simulink model "ofdm_agc_mimo"  (Simulink 7.7)
settings: Solver=VariableStepDiscrete  SolverMode=SingleTasking  StartTime=0.0  StopTime=400  RelTol=1e-3
InitFcn:
  | ofdm_agc_init
StartFcn:
  | ofdm_agc_init
values from neighbouring files (symbols this model uses):
  ltbl = ltbl(2:2049)    [ofdm_agc_init.m]
undefined symbols (not defined in the file or in its folder): gcbh, xlBlockLoadCallback, xlGetNormalizedPeriod
libraries: xbsIndex_r4 x570
(part 1 of 6)
settings Model: Creator=murphpo  LastModifiedBy=murphpo
settings OptimizationCC: InlineParams=on  InitFltsAndDblsToZero=on
settings DebuggingCC: SaveWithParameterizedLinksMsg=none  SignalResolutionControl=TryResolveAllWithWarning  MultiTaskDSMMsg=warning  MultiTaskCondExecSysMsg=none
settings RTWCC: IncludeERTFirstTime=on
settings GRTTargetCC: TargetFcnLib=ansi_tfl_tmw.mat

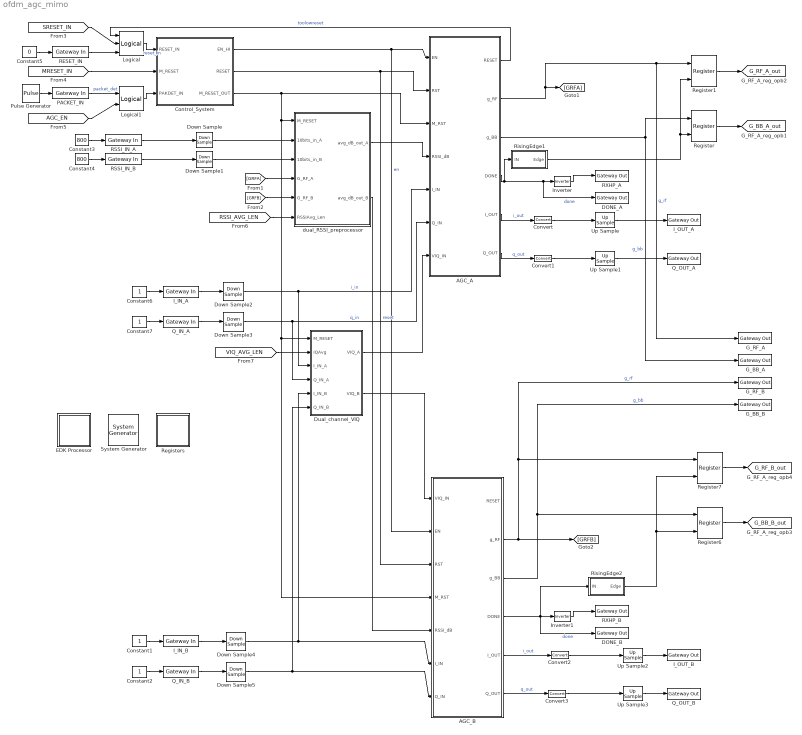
== system ofdm_agc_mimo ==
  " System Generator" : xbsIndex_r4/ System Generator  Tag=genX  SystemSampleTime=-1  xilinxfamily=virtex6  part=xc6vlx130t  speed=-1  package=ff1156  synthesis_tool=XST  clock_wrapper=Clock Enables  directory=./plb46_V6_v0  proj_type=Project Navigator  Synth_file=XST Defaults  Impl_file=ISE Defaults  testbench=off  simulink_period=1  sysclk_period=10  dcm_input_clock_period=100  incr_netlist=off  trim_vbits=Everywhere in SubSystem  dbl_ovrd=According to Block Masks  core_generation=According to Block Masks  run_coregen=off  deprecated_control=off  eval_field=0  block_type=sysgen
      settings: block_version=8.2
  AGC_A : Subsystem
  AGC_B : Subsystem
  Constant{1..2,6..7} (4 alike) : Constant
  Constant3 : Constant  Value=800
  Constant4 : Constant  Value=800
  Constant5 : Constant  Value=0
  Control_System : Subsystem
  Convert{,1..3} (4 alike) : xbsIndex_r4/Convert  gui_display_data_type=Fixed-point  arith_type="Signed  (2's comp)"  n_bits=14  bin_pt=13  float_type=Single  exp_bits=8  fraction_bits=24  quantization=Truncate  overflow=Saturate  en=off  latency=0  dbl_ovrd=off  pipeline=off  block_type=convert
      settings: xl_area=[8 0 0 15 0 0 0]  block_version=VER_STRING_GOES_HERE
  DONE_A : xbsIndex_r4/Gateway Out  inherit_from_input=off  hdl_port=on  timing_constraint=None  locs_specified=off  LOCs={}  UseAsDAC=off  DACChannel='1'  block_type=gatewayout
      settings: infoedit="Gateway out block.  Converts Xilinx fixed point inputs into ouputs of type Simulink integer, double, or fixed point.<P><P>Hardware notes:  In hardware these blocks become top level output ports or are discarded, depending on how they are configured."  xl_area=[0 0 0 0 1 0 0]  block_version=VER_STRING_GOES_HERE
  DONE_B : xbsIndex_r4/Gateway Out  inherit_from_input=off  hdl_port=on  timing_constraint=None  locs_specified=off  LOCs={}  UseAsDAC=off  DACChannel='1'  block_type=gatewayout
      settings: infoedit="Gateway out block.  Converts Xilinx fixed point inputs into ouputs of type Simulink integer, double, or fixed point.<P><P>Hardware notes:  In hardware these blocks become top level output ports or are discarded, depending on how they are configured."  xl_area=[0 0 0 0 1 0 0]  block_version=VER_STRING_GOES_HERE
  Down Sample{,1..5} (6 alike) : xbsIndex_r4/Down Sample  sample_ratio=4  sample_phase="Last Value of Frame  (most efficient)"  en=off  latency=1  dbl_ovrd=off  block_type=dsamp
      Down Sample settings: block_version=8.2.02
      Down Sample1 settings: block_version=8.2.02
      Down Sample2 settings: xl_area=[7 14 0 0 0 0 0]  block_version=VER_STRING_GOES_HERE
      Down Sample3 settings: xl_area=[7 14 0 0 0 0 0]  block_version=VER_STRING_GOES_HERE
      Down Sample4 settings: xl_area=[7 14 0 0 0 0 0]  block_version=VER_STRING_GOES_HERE
      Down Sample5 settings: xl_area=[7 14 0 0 0 0 0]  block_version=VER_STRING_GOES_HERE
  Dual_channel_VIQ : Subsystem
  EDK Processor : Subsystem  LoadFcn=xlBlockLoadCallback(gcbh);  mask(Xilinx EDK Processor Block){mode=EDK pcore generation, xmp=, MemVisToProc=<qt bgcolor="#FFFFFF"><div><img src="C:/Xilinx/13.4/ISE_DS/ISE/sysgen/data/images/registerplus.gif"> &lt;&lt;Bits_w&gt;&gt;<br></div><div><img src="C:/Xilinx/13.4/ISE_DS/ISE/sysgen/data/images/registerplus.gif"> &lt;&lt;GBB_init&gt;&gt;<br></div><div><img src="C:/Xilinx/13.4/ISE_DS/ISE/sysgen/data/images/registerplus.gif"> &lt;&lt;ADJ&gt;&gt;<br></div><div><img src="C:/Xilinx/13.4/ISE_DS/ISE/sysgen/data/images/registerplus.gif"> &lt;&lt;DCO_IIR_Coef_FB&gt;&gt;<br></div><div><img src="C:/Xilinx/13.4/ISE_DS/ISE/sysgen/data/images/registerplus.gif"> &lt;&lt;Thresholds&gt;&gt;<br></div><div><img src="C:/Xilinx/13.4/ISE_DS/ISE/sysgen/data/images/registerplus.gif"> &lt;&lt;Timing&gt;&gt;<br></div><div><img src="C:/Xilinx/13.4/ISE_DS/ISE/sysgen/data/images/registerplus.gif"> &lt;&lt;DCO_IIR_Coef_Gain&gt;&gt;<br></div><div><img src="C:/Xilinx/13.4/ISE_DS/ISE/sysgen/data/images/registerplus.gif"> &lt;&lt;AVG_LEN&gt;&gt;<br></div><div><img src="C:/Xilinx/13.4/ISE_DS/ISE/sysgen/data/images/registerplus.gif"> &lt;&lt;AGC_EN&gt;&gt;<br></div><div><img src="C:/Xilinx/13.4/ISE_DS/ISE/sysgen/data/images/registerplus.gif"> &lt;&lt;DCO_Timing&gt;&gt;<br></div><div><img src="C:/Xilinx/13.4/ISE_DS/ISE/sysgen/data/images/registerplus.gif"> &lt;&lt;T_dB&gt;&gt;<br></div><div><img src="C:/Xilinx/13.4/ISE_DS/ISE/sysgen/data/images/registerplus.gif"> &lt;&lt;MRESET_IN&gt;&gt;<br></div><div><img src="C:/Xilinx/13.4/ISE_DS/ISE/sysgen/data/images/registerplus.gif"> &lt;&lt;SRESET_IN&gt;&gt;<br></div><div><img src="C:/Xilinx/13.4/ISE_DS/ISE/sysgen/data/images/registerplus.gif"> &lt;&lt;GRF_A&gt;&gt;<br></div><div><img src="C:/Xilinx/13.4/ISE_DS/ISE/sysgen/data/images/registerplus.gif"> &lt;&lt;GRF_B&gt;&gt;<br></div><div><img src="C:/Xilinx/13.4/ISE_DS/ISE/sysgen/data/images/registerplus.gif"> &lt;&lt;GBB_B&gt;&gt;<br></div><div><img src="C:/Xilinx/13.4/ISE_DS/ISE/sysgen/data/images/registerplus.gif"> &lt;&lt;GBB_A&gt;&gt;<br></div><div><img src="C:/Xilinx/13.4/ISE_DS/ISE/sysgen/data/images/registerplus.gif"> &lt;&lt;Bits_r&gt;&gt;<br></div></qt>, AvailableMemories=<empty>, portInterfaceTable={'exposed'=>[],'portdir'=>[],'portname'=>[],'shortname'=>[]}, bus_type_sgadvanced=, bus_type=PLB, baseaddr=0x80000000, baseaddr_lock_sgadvanced=, baseaddr_lock=off, dual_clock_sgadvanced=, dual_clock=on, reg_readback_sgadvanced=, reg_readback=on, ucf_file=, inheritDeviceType_sgadvanced=, inheritDeviceType=off, elf_file=, codebug_sgadvanced=, codebug=on, clock_name=plb, internalPortList={}, resetPolarity=0, memxtable={'mladdr'=>[0.00000000000000000,1.00000000000000000,2.00000000000000000,3.00000000000000000,4.00000000000000000,5.00000000000000000,6.00000000000000000,7.00000000000000000,8.00000000000000000,9.00000000000000000,10.00000000000000000,11.00000000000000000,12.00000000000000000,0.00000000000000000,1.00000000000000000,2.00000000000000000,3.00000000000000000,4.00000000000000000],'mlist'=>['ofdm_agc_mimo/Registers/Read-Write Register/From Register','ofdm_agc_mimo/Registers/From Register9','ofdm_agc_mimo/Registers/From Register8','ofdm_agc_mimo/Registers/From Register7','ofdm_agc_mimo/Registers/From Register6','ofdm_agc_mimo/Registers/From Register5','ofdm_agc_mimo/Registers/From Register4','ofdm_agc_mimo/Registers/From Register3','ofdm_agc_mimo/Registers/From Register2','ofdm_agc_mimo/Registers/From Register11','ofdm_agc_mimo/Registers/From Register10','ofdm_agc_mimo/Registers/From Register1','ofdm_agc_mimo/Registers/From Register','ofdm_agc_mimo/Registers/To Register3','ofdm_agc_mimo/Registers/To Register2','ofdm_agc_mimo/Registers/To Register1','ofdm_agc_mimo/Registers/To Register','ofdm_agc_mimo/Registers/Read-Write Register/To Register'],'mlname'=>['\\'Bits_w\\'','\\'GBB_init\\'','\\'ADJ\\'','\\'DCO_IIR_Coef_FB\\'','\\'Thresholds\\'','\\'Timing\\'','\\'DCO_IIR_Coef_Gain\\'','\\'AVG_LEN\\'','\\'AGC_EN\\'','\\'DCO_Timing\\'','\\'T_dB\\'','\\'MRESET_IN\\'','\\'SRESET_IN\\'','\\'GRF_A\\'','\\'GRF_B\\'','\\'GBB_B\\'','\\'GBB_A\\'','\\'Bits_r\\''],'mlstate'=>[0.00000000000000000,0.00000000000000000,0.00000000000000000,0.00000000000000000,0.00000000000000000,0.00000000000000000,0.00000000000000000,0.00000000000000000,0.00000000000000000,0.00000000000000000,0.00000000000000000,0.00000000000000000,0.00000000000000000,0.00000000000000000,0.00000000000000000,0.00000000000000000,0.00000000000000000,0.00000000000000000]}, procinfo={}, memmapdirty=off, blockname=, xpsintstyle=default, has_advanced_control=0, sggui_pos=-1,-1,-1,-1, block_type=edkprocessor, block_version=2.7, sg_icon_stat=55,55,-1,-1,white,blue,0,07734,right,,[ ],[ ], sg_mask_display=|, sg_list_contents={'table'=>{'AvailableMemories'=>'popup(<empty>)'}}, sg_blockgui_xml=}
      mask sg_mask_display=|
      | fprintf('','COMMENT: begin icon graphics');
      | patch([0 55 55 0 0 ],[0 0 55 55 0 ],[0.77 0.82 0.91 ]);
      | plot([0 55 55 0 0 ],[0 0 55 55 0 ]);
      | patch([11.425 21.54 28.54 35.54 42.54 28.54 18.425 11.425 ],[34.77 34.77 41.77 34.77 41.77 41.77 41.77 34.77 ],[1 1 1 ]);
      | patch([18.425 28.54 21.54 11.425 18.425 ],[27.77 27.77 34.77 34.77 27.77 ],[0.931 0.946 0.973 ]);
      | patch([11.425 21.54 28.54 18.425 11.425 ],[20.77 20.77 27.77 27.77 20.77 ],[1 1 1 ]);
      | patch([18.425 42.54 35.54 28.54 21.54 11.425 18.425 ],[13.77 13.77 20.77 13.77 20.77 20.77 13.77 ],[0.931 0.946 0.973 ]);
      | fprintf('','COMMENT: end icon graphics');
      | fprintf('','COMMENT: begin icon text');
      | fprintf('','COMMENT: end icon text');
      mask prompts: mode "Configure Processor for"; xmp "XPS Project"; MemVisToProc ""; AvailableMemories "Available Memories"; portInterfaceTable ""; bus_type_sgadvanced ""; bus_type "Bus Type"; baseaddr "Base Address"; baseaddr_lock_sgadvanced ""; baseaddr_lock "Lock"; dual_clock_sgadvanced ""; dual_clock "Dual Clocks"; reg_readback_sgadvanced ""; reg_readback "Register Read-Back"; ucf_file "Constraint File"; inheritDeviceType_sgadvanced ""; inheritDeviceType "Inherit Device Type"; elf_file "Initial Program"; codebug_sgadvanced ""; codebug "Enable Co-Debug with Xilinx SDK (Beta)"; clock_name ""; internalPortList ""; resetPolarity ""; memxtable ""; procinfo ""; memmapdirty ""; blockname ""; xpsintstyle ""; has_advanced_control ""; sggui_pos ""; block_type ""; block_version ""; sg_icon_stat ""; sg_mask_display ""; sg_list_contents ""; sg_blockgui_xml ""
      mask help: Xilinx EDK Processor
      mask init:
      | try
      |   tmp_gcb = gcb;
      |   tmp_gcbh = gcbh;
      |   if (strcmp('SysGenIndex',get_param(bdroot(tmp_gcbh),'tag')) && ~isempty(regexp(bdroot(tmp_gcb), '^xbs', 'once')))
      |     return;
      |   end;
      |   xlMungeMaskParams;
      | 
      |   block_type='edkprocessor';
      | 
      |   serialized_declarations = '{''block_type''=>''String''}';
      |   xledkprocessor_init();
      |   ptable_ = xlblockprep(get_param(tmp_gcb, 'MaskWSVariables'));
      |   try
      |     xlBlockMoveCallback(tmp_gcbh);
      |   catch 
      |      clear global xl_updateicon_recursion_guard;
      |   end;
      | catch
      |   global dbgsysgen;
      |   if(~isempty(dbgsysgen) && dbgsysgen)
      |     e = regexprep(lasterr, '\n', '\nError: ');
      |     disp(['Error: While running MaskInit code on block ' tmp_gcb ': ' e]);
      |     error(e);
      |   end
      | end
      settings: CopyFcn=xlProcBlockCopyCallback(gcbh);xlBlockMoveCallback(gcbh);  DeleteFcn=xlDestroyGui(gcbh);  ModelCloseFcn=xlDestroyGui(gcbh);  PreSaveFcn=xlBlockPreSaveCallback(gcbh);  PostSaveFcn=xlBlockPostSaveCallback(gcbh);  DestroyFcn=xlDestroyGui(gcbh);  OpenFcn=bh=gcbh;xlProcBlockCallbacks('populatesharedmemorylistbox',bh);xlOpenGui(bh, 'edkprocessor_gui.xml', @xlProcBlockEnablement, @xlProcBlockAction);  CloseFcn=xlDestroyGui(gcbh);  MoveFcn=xlBlockMoveCallback(gcbh);
      mask Help: eval('');xlDoc('-book','sysgen','-topic','EDK_Processor');
      mask StyleString: popup(EDK pcore generation|HDL netlisting),edit,edit,edit,edit,edit,popup(AXI|PLB),edit,edit,checkbox,edit,checkbox,edit,checkbox,edit,edit,checkbox,edit,edit,checkbox,edit,edit,edit,edit,edit,edit,edit,edit,edit,edit,edit,edit,edit,edit,edit,edit
      mask Display:
      | fprintf('','COMMENT: begin icon graphics');
      | patch([0 55 55 0 0 ],[0 0 55 55 0 ],[0.77 0.82 0.91 ]);
      | plot([0 55 55 0 0 ],[0 0 55 55 0 ]);
      | patch([11.425 21.54 28.54 35.54 42.54 28.54 18.425 11.425 ],[34.77 34.77 41.77 34.77 41.77 41.77 41.77 34.77 ],[1 1 1 ]);
      | patch([18.425 28.54 21.54 11.425 18.425 ],[27.77 27.77 34.77 34.77 27.77 ],[0.931 0.946 0.973 ]);
      | patch([11.425 21.54 28.54 18.425 11.425 ],[20.77 20.77 27.77 27.77 20.77 ],[1 1 1 ]);
      | patch([18.425 42.54 35.54 28.54 21.54 11.425 18.425 ],[13.77 13.77 20.77 13.77 20.77 20.77 13.77 ],[0.931 0.946 0.973 ]);
      | fprintf('','COMMENT: end icon graphics');
      | fprintf('','COMMENT: begin icon text');
      | disp('');
      | 
      | fprintf('','COMMENT: end icon text');
  G_BB_A : xbsIndex_r4/Gateway Out  inherit_from_input=off  hdl_port=on  timing_constraint=None  locs_specified=off  LOCs={}  UseAsDAC=off  DACChannel='1'  block_type=gatewayout
      settings: infoedit="Gateway out block.  Converts Xilinx fixed point inputs into ouputs of type Simulink integer, double, or fixed point.<P><P>Hardware notes:  In hardware these blocks become top level output ports or are discarded, depending on how they are configured."  xl_area=[0 0 0 0 5 0 0]  block_version=VER_STRING_GOES_HERE
  G_BB_B : xbsIndex_r4/Gateway Out  inherit_from_input=off  hdl_port=on  timing_constraint=None  locs_specified=off  LOCs={}  UseAsDAC=off  DACChannel='1'  block_type=gatewayout
      settings: infoedit="Gateway out block.  Converts Xilinx fixed point inputs into ouputs of type Simulink integer, double, or fixed point.<P><P>Hardware notes:  In hardware these blocks become top level output ports or are discarded, depending on how they are configured."  xl_area=[0 0 0 0 5 0 0]  block_version=VER_STRING_GOES_HERE
  G_RF_A : xbsIndex_r4/Gateway Out  inherit_from_input=off  hdl_port=on  timing_constraint=None  locs_specified=off  LOCs={}  UseAsDAC=off  DACChannel='1'  block_type=gatewayout
      settings: infoedit="Gateway out block.  Converts Xilinx fixed point inputs into ouputs of type Simulink integer, double, or fixed point.<P><P>Hardware notes:  In hardware these blocks become top level output ports or are discarded, depending on how they are configured."  xl_area=[0 0 0 0 2 0 0]  block_version=VER_STRING_GOES_HERE
  G_RF_B : xbsIndex_r4/Gateway Out  inherit_from_input=off  hdl_port=on  timing_constraint=None  locs_specified=off  LOCs={}  UseAsDAC=off  DACChannel='1'  block_type=gatewayout
      settings: infoedit="Gateway out block.  Converts Xilinx fixed point inputs into ouputs of type Simulink integer, double, or fixed point.<P><P>Hardware notes:  In hardware these blocks become top level output ports or are discarded, depending on how they are configured."  xl_area=[0 0 0 0 2 0 0]  block_version=VER_STRING_GOES_HERE
  I_IN_A : xbsIndex_r4/Gateway In  gui_display_data_type=Fixed-point  arith_type="Signed  (2's comp)"  n_bits=14  bin_pt=13  preci_type=Single  exp_width=8  frac_width=24  quantization="Round  (unbiased: +/- Inf)"  overflow=Saturate  period=1  dbl_ovrd=off  timing_constraint=None  locs_specified=off  LOCs={}  inherit_from_input=off  UseAsADC=off  ADCChannel='1'  hdl_port=on  block_type=gatewayin
      settings: infoedit="Gateway in block.  Converts inputs of type Simulink integer, double and fixed point to  Xilinx fixed point type.<P><P>Hardware notes:  In hardware these blocks become top level input ports."  xl_area=[0 0 0 0 14 0 0]  block_version=VER_STRING_GOES_HERE
  I_IN_B : xbsIndex_r4/Gateway In  gui_display_data_type=Fixed-point  arith_type="Signed  (2's comp)"  n_bits=14  bin_pt=13  preci_type=Single  exp_width=8  frac_width=24  quantization="Round  (unbiased: +/- Inf)"  overflow=Saturate  period=1  dbl_ovrd=off  timing_constraint=None  locs_specified=off  LOCs={}  inherit_from_input=off  UseAsADC=off  ADCChannel='1'  hdl_port=on  block_type=gatewayin
      settings: infoedit="Gateway in block.  Converts inputs of type Simulink integer, double and fixed point to  Xilinx fixed point type.<P><P>Hardware notes:  In hardware these blocks become top level input ports."  xl_area=[0 0 0 0 14 0 0]  block_version=VER_STRING_GOES_HERE
  I_OUT_A : xbsIndex_r4/Gateway Out  inherit_from_input=off  hdl_port=on  timing_constraint=None  locs_specified=off  LOCs={}  UseAsDAC=off  DACChannel='1'  block_type=gatewayout
      settings: infoedit="Gateway out block.  Converts Xilinx fixed point inputs into ouputs of type Simulink integer, double, or fixed point.<P><P>Hardware notes:  In hardware these blocks become top level output ports or are discarded, depending on how they are configured."  xl_area=[0 0 0 0 14 0 0]  block_version=VER_STRING_GOES_HERE
  I_OUT_B : xbsIndex_r4/Gateway Out  inherit_from_input=off  hdl_port=on  timing_constraint=None  locs_specified=off  LOCs={}  UseAsDAC=off  DACChannel='1'  block_type=gatewayout
      settings: infoedit="Gateway out block.  Converts Xilinx fixed point inputs into ouputs of type Simulink integer, double, or fixed point.<P><P>Hardware notes:  In hardware these blocks become top level output ports or are discarded, depending on how they are configured."  xl_area=[0 0 0 0 14 0 0]  block_version=VER_STRING_GOES_HERE
  Inverter : xbsIndex_r4/Inverter  en=off  latency=0  dbl_ovrd=off  block_type=inv
      settings: xl_area=[0 0 0 0 0 0 0]  block_version=VER_STRING_GOES_HERE
  Inverter1 : xbsIndex_r4/Inverter  en=off  latency=0  dbl_ovrd=off  block_type=inv
      settings: xl_area=[0 0 0 0 0 0 0]  block_version=VER_STRING_GOES_HERE
  Logical : xbsIndex_r4/Logical  logical_function=OR  inputs=3  en=off  latency=0  precision=Full  arith_type=Unsigned  n_bits=16  bin_pt=0  align_bp=on  dbl_ovrd=off  block_type=logical
      settings: xl_area=[1 0 0 1 0 0 0]  block_version=VER_STRING_GOES_HERE
  Logical1 : xbsIndex_r4/Logical  logical_function=AND  inputs=2  en=off  latency=0  precision=Full  arith_type=Unsigned  n_bits=16  bin_pt=0  align_bp=on  dbl_ovrd=off  block_type=logical
      settings: xl_area=[1 0 0 1 0 0 0]  block_version=VER_STRING_GOES_HERE
  PACKET_IN : xbsIndex_r4/Gateway In  gui_display_data_type=Fixed-point  arith_type=Boolean  n_bits=10  bin_pt=0  preci_type=Single  exp_width=8  frac_width=24  quantization="Round  (unbiased: +/- Inf)"  overflow=Saturate  period=1  dbl_ovrd=off  timing_constraint=None  locs_specified=off  LOCs={}  inherit_from_input=off  UseAsADC=off  ADCChannel='1'  hdl_port=on  block_type=gatewayin
      settings: infoedit="Gateway in block.  Converts inputs of type Simulink integer, double and fixed point to  Xilinx fixed point type.<P><P>Hardware notes:  In hardware these blocks become top level input ports."  xl_area=[0 0 0 0 1 0 0]  block_version=VER_STRING_GOES_HERE
  Pulse Generator : DiscretePulseGenerator  Period=1e5  PulseWidth=4  PhaseDelay=5
  Q_IN_A : xbsIndex_r4/Gateway In  gui_display_data_type=Fixed-point  arith_type="Signed  (2's comp)"  n_bits=14  bin_pt=13  preci_type=Single  exp_width=8  frac_width=24  quantization="Round  (unbiased: +/- Inf)"  overflow=Saturate  period=1  dbl_ovrd=off  timing_constraint=None  locs_specified=off  LOCs={}  inherit_from_input=off  UseAsADC=off  ADCChannel='1'  hdl_port=on  block_type=gatewayin
      settings: infoedit="Gateway in block.  Converts inputs of type Simulink integer, double and fixed point to  Xilinx fixed point type.<P><P>Hardware notes:  In hardware these blocks become top level input ports."  xl_area=[0 0 0 0 14 0 0]  block_version=VER_STRING_GOES_HERE
  Q_IN_B : xbsIndex_r4/Gateway In  gui_display_data_type=Fixed-point  arith_type="Signed  (2's comp)"  n_bits=14  bin_pt=13  preci_type=Single  exp_width=8  frac_width=24  quantization="Round  (unbiased: +/- Inf)"  overflow=Saturate  period=1  dbl_ovrd=off  timing_constraint=None  locs_specified=off  LOCs={}  inherit_from_input=off  UseAsADC=off  ADCChannel='1'  hdl_port=on  block_type=gatewayin
      settings: infoedit="Gateway in block.  Converts inputs of type Simulink integer, double and fixed point to  Xilinx fixed point type.<P><P>Hardware notes:  In hardware these blocks become top level input ports."  xl_area=[0 0 0 0 14 0 0]  block_version=VER_STRING_GOES_HERE
  Q_OUT_A : xbsIndex_r4/Gateway Out  inherit_from_input=off  hdl_port=on  timing_constraint=None  locs_specified=off  LOCs={}  UseAsDAC=off  DACChannel='1'  block_type=gatewayout
      settings: infoedit="Gateway out block.  Converts Xilinx fixed point inputs into ouputs of type Simulink integer, double, or fixed point.<P><P>Hardware notes:  In hardware these blocks become top level output ports or are discarded, depending on how they are configured."  xl_area=[0 0 0 0 14 0 0]  block_version=VER_STRING_GOES_HERE
  Q_OUT_B : xbsIndex_r4/Gateway Out  inherit_from_input=off  hdl_port=on  timing_constraint=None  locs_specified=off  LOCs={}  UseAsDAC=off  DACChannel='1'  block_type=gatewayout
      settings: infoedit="Gateway out block.  Converts Xilinx fixed point inputs into ouputs of type Simulink integer, double, or fixed point.<P><P>Hardware notes:  In hardware these blocks become top level output ports or are discarded, depending on how they are configured."  xl_area=[0 0 0 0 14 0 0]  block_version=VER_STRING_GOES_HERE
  RESET_IN : xbsIndex_r4/Gateway In  gui_display_data_type=Fixed-point  arith_type=Boolean  n_bits=10  bin_pt=0  preci_type=Single  exp_width=8  frac_width=24  quantization="Round  (unbiased: +/- Inf)"  overflow=Saturate  period=1  dbl_ovrd=off  timing_constraint=None  locs_specified=off  LOCs={}  inherit_from_input=off  UseAsADC=off  ADCChannel='1'  hdl_port=on  block_type=gatewayin
      settings: infoedit="Gateway in block.  Converts inputs of type Simulink integer, double and fixed point to  Xilinx fixed point type.<P><P>Hardware notes:  In hardware these blocks become top level input ports."  xl_area=[0 0 0 0 1 0 0]  block_version=VER_STRING_GOES_HERE
  RSSI_IN_A : xbsIndex_r4/Gateway In  gui_display_data_type=Fixed-point  arith_type=Unsigned  n_bits=10  bin_pt=0  preci_type=Single  exp_width=8  frac_width=24  quantization="Round  (unbiased: +/- Inf)"  overflow=Saturate  period=1  dbl_ovrd=off  timing_constraint=None  locs_specified=off  LOCs={}  inherit_from_input=off  UseAsADC=off  ADCChannel='1'  hdl_port=on  block_type=gatewayin
      settings: infoedit="Gateway in block.  Converts inputs of type Simulink integer, double and fixed point to  Xilinx fixed point type.<P><P>Hardware notes:  In hardware these blocks become top level input ports."  xl_area=[0 0 0 0 10 0 0]  block_version=VER_STRING_GOES_HERE
  RSSI_IN_B : xbsIndex_r4/Gateway In  gui_display_data_type=Fixed-point  arith_type=Unsigned  n_bits=10  bin_pt=0  preci_type=Single  exp_width=8  frac_width=24  quantization="Round  (unbiased: +/- Inf)"  overflow=Saturate  period=1  dbl_ovrd=off  timing_constraint=None  locs_specified=off  LOCs={}  inherit_from_input=off  UseAsADC=off  ADCChannel='1'  hdl_port=on  block_type=gatewayin
      settings: infoedit="Gateway in block.  Converts inputs of type Simulink integer, double and fixed point to  Xilinx fixed point type.<P><P>Hardware notes:  In hardware these blocks become top level input ports."  xl_area=[0 0 0 0 10 0 0]  block_version=VER_STRING_GOES_HERE
  RXHP_A : xbsIndex_r4/Gateway Out  inherit_from_input=off  hdl_port=on  timing_constraint=None  locs_specified=off  LOCs={}  UseAsDAC=off  DACChannel='1'  block_type=gatewayout
      settings: infoedit="Gateway out block.  Converts Xilinx fixed point inputs into ouputs of type Simulink integer, double, or fixed point.<P><P>Hardware notes:  In hardware these blocks become top level output ports or are discarded, depending on how they are configured."  xl_area=[0 0 0 0 1 0 0]  block_version=VER_STRING_GOES_HERE
  RXHP_B : xbsIndex_r4/Gateway Out  inherit_from_input=off  hdl_port=on  timing_constraint=None  locs_specified=off  LOCs={}  UseAsDAC=off  DACChannel='1'  block_type=gatewayout
      settings: infoedit="Gateway out block.  Converts Xilinx fixed point inputs into ouputs of type Simulink integer, double, or fixed point.<P><P>Hardware notes:  In hardware these blocks become top level output ports or are discarded, depending on how they are configured."  xl_area=[0 0 0 0 1 0 0]  block_version=VER_STRING_GOES_HERE
  Register{,1,6..7} (4 alike) : xbsIndex_r4/Register  init=0  rst=off  en=on  dbl_ovrd=off  block_type=register
      Register settings: xl_area=[3 5 0 0 0 0 0]  block_version=VER_STRING_GOES_HERE
      Register1 settings: xl_area=[1 2 0 0 0 0 0]  block_version=VER_STRING_GOES_HERE
      Register6 settings: xl_area=[3 5 0 0 0 0 0]  block_version=VER_STRING_GOES_HERE
      Register7 settings: xl_area=[1 2 0 0 0 0 0]  block_version=VER_STRING_GOES_HERE
  Registers : Subsystem
  RisingEdge1 : Subsystem
  RisingEdge2 : Subsystem
  Up Sample{,1..3} (4 alike) : xbsIndex_r4/Up Sample  sample_ratio=4  copy_samples=on  en=off  latency=0  dbl_ovrd=off  block_type=usamp
      settings: infoedit="Up samples input data.  Inserted values  can be zeros or copies of the most recent input sample.<P><P>Hardware notes: No hardware is needed if inserted values are copies of the input sample; otherwise, a mux and single bit flip-flop are used."  block_version=8.2.02
  dual_RSSI_preprocessor : Subsystem
  tag scope: G_BB_A_out=global, G_BB_B_out=global, G_RF_A_out=global, G_RF_B_out=global
  wires:
  AGC_A/2(g_RF) -> [GRFA], Register1/1, G_RF_A/1  "g_rf"
  Control_System/1(EN_HI) -> AGC_A/1(EN), AGC_B/2(EN)  "en"
  Control_System/2(RESET) -> AGC_A/2(RST), AGC_B/3(RST)  "reset"
  Control_System/3(M_RESET_OUT) -> AGC_A/3(M_RST), Dual_channel_VIQ/1(M_RESET), AGC_B/4(M_RST), dual_RSSI_preprocessor/1(M_RESET)
  Down Sample2/1 -> AGC_A/5(I_IN), Dual_channel_VIQ/3(I_IN_A)  "i_in"
  Down Sample3/1 -> AGC_A/6(Q_IN), Dual_channel_VIQ/4(Q_IN_A)  "q_in"
  I_IN_A/1 -> Down Sample2/1
  Q_IN_A/1 -> Down Sample3/1
  AGC_A/5(I_OUT) -> Convert/1  "i_out"
  AGC_A/6(Q_OUT) -> Convert1/1  "q_out"
  Inverter/1 -> RXHP_A/1
  Logical/1 -> Control_System/1(RESET_IN)  "reset_in"
  AGC_A/1(RESET) -> Logical/1  "toolowreset"
  Constant5/1 -> RESET_IN/1
  Pulse Generator/1 -> PACKET_IN/1
  Constant3/1 -> RSSI_IN_A/1
  Constant6/1 -> I_IN_A/1
  Constant7/1 -> Q_IN_A/1
  RESET_IN/1 -> Logical/3
  PACKET_IN/1 -> Logical1/1  "packet_det"
  Logical1/1 -> Control_System/3(PAKDET_IN)
  Convert/1 -> Up Sample/1
  Convert1/1 -> Up Sample1/1
  AGC_A/4(DONE) -> DONE_A/1, Inverter/1, RisingEdge1/1(IN)  "done"
  AGC_A/3(g_BB) -> Register/1, G_BB_A/1  "g_bb"
  RisingEdge1/1(Edge) -> Register/2, Register1/2
  Constant4/1 -> RSSI_IN_B/1
  AGC_B/2(g_RF) -> [GRFB], Register7/1, G_RF_B/1  "g_rf"
  Constant1/1 -> I_IN_B/1
  Constant2/1 -> Q_IN_B/1
  AGC_B/5(I_OUT) -> Convert2/1  "i_out"
  AGC_B/6(Q_OUT) -> Convert3/1  "q_out"
  Inverter1/1 -> RXHP_B/1
  Convert2/1 -> Up Sample2/1
  Convert3/1 -> Up Sample3/1
  AGC_B/4(DONE) -> Inverter1/1, DONE_B/1, RisingEdge2/1(IN)  "done"
  Down Sample4/1 -> Dual_channel_VIQ/5(I_IN_B), AGC_B/6(I_IN)
  Down Sample5/1 -> Dual_channel_VIQ/6(Q_IN_B), AGC_B/7(Q_IN)
  Dual_channel_VIQ/2(VIQ_B) -> AGC_B/1(VIQ_IN)
  Dual_channel_VIQ/1(VIQ_A) -> AGC_A/7(VIQ_IN)
  AGC_B/3(g_BB) -> Register6/1, G_BB_B/1  "g_bb"
  RSSI_IN_A/1 -> Down Sample/1
  RSSI_IN_B/1 -> Down Sample1/1
  [GRFA] -> dual_RSSI_preprocessor/4(G_RF_A)
  [GRFB] -> dual_RSSI_preprocessor/5(G_RF_B)
  dual_RSSI_preprocessor/1(avg_dB_out_A) -> AGC_A/4(RSSI_dB)
  dual_RSSI_preprocessor/2(avg_dB_out_B) -> AGC_B/5(RSSI_dB)
  RisingEdge2/1(Edge) -> Register6/2, Register7/2
  [AGC_EN] -> Logical1/2
  [MRESET_IN] -> Control_System/2(M_RESET)
  [SRESET_IN] -> Logical/2
  Register/1 -> [G_BB_A_out]
  Register6/1 -> [G_BB_B_out]
  Register1/1 -> [G_RF_A_out]
  Register7/1 -> [G_RF_B_out]
  [RSSI_AVG_LEN] -> dual_RSSI_preprocessor/6(RSSIAvg_Len)
  [VIQ_AVG_LEN] -> Dual_channel_VIQ/2(IQAvg)
  Down Sample/1 -> dual_RSSI_preprocessor/2(10bits_in_A)
  Down Sample1/1 -> dual_RSSI_preprocessor/3(10bits_in_B)
  Up Sample/1 -> I_OUT_A/1
  Up Sample1/1 -> Q_OUT_A/1
  Up Sample2/1 -> I_OUT_B/1
  Up Sample3/1 -> Q_OUT_B/1
  I_IN_B/1 -> Down Sample4/1
  Q_IN_B/1 -> Down Sample5/1

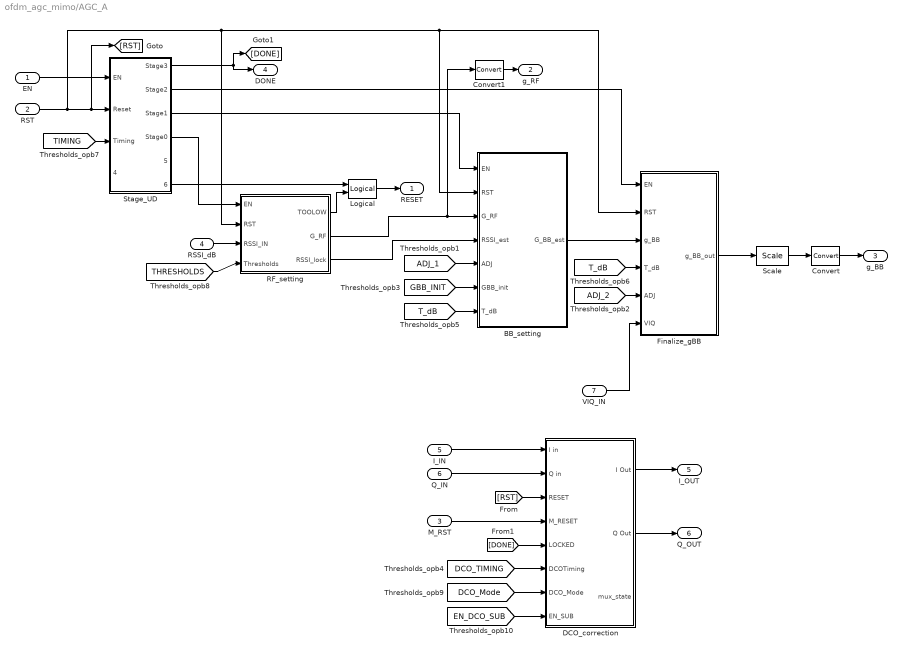
== system ofdm_agc_mimo/AGC_A ==
  EN : Inport
  RST : Inport  Port=2
  M_RST : Inport  Port=3
  RSSI_dB : Inport  Port=4
  I_IN : Inport  Port=5
  Q_IN : Inport  Port=6
  VIQ_IN : Inport  Port=7
  BB_setting : Subsystem
  Convert : xbsIndex_r4/Convert  gui_display_data_type=Fixed-point  arith_type=Unsigned  n_bits=5  bin_pt=0  float_type=Single  exp_bits=8  fraction_bits=24  quantization="Round  (unbiased: +/- Inf)"  overflow=Saturate  en=off  latency=0  dbl_ovrd=off  pipeline=off  block_type=convert
      settings: xl_area=[9 0 0 18 0 0 0]  block_version=VER_STRING_GOES_HERE
  Convert1 : xbsIndex_r4/Convert  gui_display_data_type=Fixed-point  arith_type=Unsigned  n_bits=2  bin_pt=0  float_type=Single  exp_bits=8  fraction_bits=24  quantization=Truncate  overflow=Wrap  en=off  latency=0  dbl_ovrd=off  pipeline=off  block_type=convert
      settings: xl_area=[0 0 0 0 0 0 0]  block_version=VER_STRING_GOES_HERE
  DCO_correction : Subsystem
  Finalize_gBB : Subsystem
  Logical : xbsIndex_r4/Logical  logical_function=OR  inputs=2  en=off  latency=0  precision=Full  arith_type=Unsigned  n_bits=16  bin_pt=0  align_bp=on  dbl_ovrd=off  block_type=logical
      settings: xl_area=[1 0 0 1 0 0 0]  block_version=VER_STRING_GOES_HERE
  RF_setting : Subsystem
  Scale : xbsIndex_r4/Scale  scale_factor=-1  dbl_ovrd=off  block_type=scale
      settings: infoedit=Scales input by a power of two by adjusting the binary point position.<P><P>Hardware notes: In hardware this block costs nothing.  block_version=VER_STRING_GOES_HERE
  Stage_UD : Subsystem
  RESET : Outport
  g_RF : Outport  Port=2
  g_BB : Outport  Port=3
  DONE : Outport  Port=4
  I_OUT : Outport  Port=5
  Q_OUT : Outport  Port=6
  wires:
  Finalize_gBB/1(g_BB_out) -> Scale/1
  Stage_UD/1(Stage3) -> [DONE], DONE/1
  RSSI_dB/1 -> RF_setting/3(RSSI_IN)
  M_RST/1 -> DCO_correction/4(M_RESET)
  Q_IN/1 -> DCO_correction/2(Q in)
  I_IN/1 -> DCO_correction/1(I in)
  EN/1 -> Stage_UD/1(EN)
  RST/1 -> RF_setting/2(RST), Finalize_gBB/2(RST), BB_setting/2(RST), Stage_UD/2(Reset), [RST]
  Stage_UD/2(Stage2) -> Finalize_gBB/1(EN)
  BB_setting/1(G_BB_est) -> Finalize_gBB/3(g_BB)
  RF_setting/2(G_RF) -> BB_setting/3(G_RF), Convert1/1
  Stage_UD/3(Stage1) -> BB_setting/1(EN)
  Stage_UD/4(Stage0) -> RF_setting/1(EN)
  DCO_correction/1(I Out) -> I_OUT/1
  DCO_correction/2(Q Out) -> Q_OUT/1
  Scale/1 -> Convert/1
  Convert/1 -> g_BB/1
  Convert1/1 -> g_RF/1
  [RST] -> DCO_correction/3(RESET)
  [DONE] -> DCO_correction/5(LOCKED)
  [DCO_Mode] -> DCO_correction/7(DCO_Mode)
  [EN_DCO_SUB] -> DCO_correction/8(EN_SUB)
  [ADJ_1] -> BB_setting/5(ADJ)
  RF_setting/3(RSSI_lock) -> BB_setting/4(RSSI_est)
  Logical/1 -> RESET/1
  RF_setting/1(TOOLOW) -> Logical/2
  Stage_UD/6(TOreset) -> Logical/1
  VIQ_IN/1 -> Finalize_gBB/6(VIQ)
  [DCO_TIMING] -> DCO_correction/6(DCOTiming)
  [THRESHOLDS] -> RF_setting/4(Thresholds)
  [TIMING] -> Stage_UD/3(Timing)
  [ADJ_2] -> Finalize_gBB/5(ADJ)
  [GBB_INIT] -> BB_setting/6(GBB_init)
  [T_dB] -> BB_setting/7(T_dB)
  [T_dB] -> Finalize_gBB/4(T_dB)

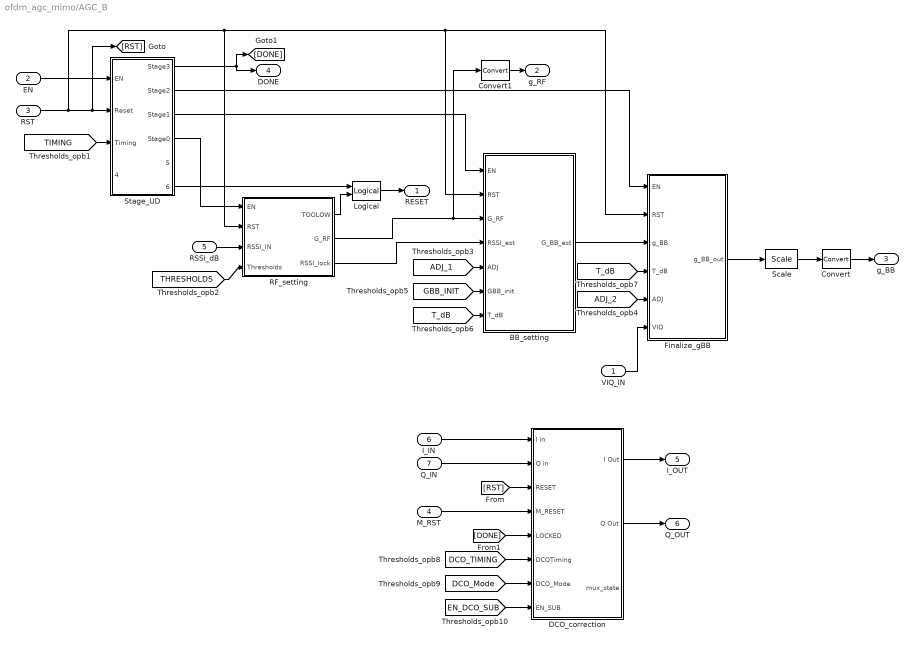
== system ofdm_agc_mimo/AGC_B ==
  VIQ_IN : Inport
  EN : Inport  Port=2
  RST : Inport  Port=3
  M_RST : Inport  Port=4
  RSSI_dB : Inport  Port=5
  I_IN : Inport  Port=6
  Q_IN : Inport  Port=7
  BB_setting : Subsystem
  Convert : xbsIndex_r4/Convert  gui_display_data_type=Fixed-point  arith_type=Unsigned  n_bits=5  bin_pt=0  float_type=Single  exp_bits=8  fraction_bits=24  quantization="Round  (unbiased: +/- Inf)"  overflow=Saturate  en=off  latency=0  dbl_ovrd=off  pipeline=off  block_type=convert
      settings: xl_area=[9 0 0 18 0 0 0]  block_version=VER_STRING_GOES_HERE
  Convert1 : xbsIndex_r4/Convert  gui_display_data_type=Fixed-point  arith_type=Unsigned  n_bits=2  bin_pt=0  float_type=Single  exp_bits=8  fraction_bits=24  quantization=Truncate  overflow=Wrap  en=off  latency=0  dbl_ovrd=off  pipeline=off  block_type=convert
      settings: xl_area=[0 0 0 0 0 0 0]  block_version=VER_STRING_GOES_HERE
  DCO_correction : Subsystem
  Finalize_gBB : Subsystem
  Logical : xbsIndex_r4/Logical  logical_function=OR  inputs=2  en=off  latency=0  precision=Full  arith_type=Unsigned  n_bits=16  bin_pt=0  align_bp=on  dbl_ovrd=off  block_type=logical
      settings: xl_area=[1 0 0 1 0 0 0]  block_version=VER_STRING_GOES_HERE
  RF_setting : Subsystem
  Scale : xbsIndex_r4/Scale  scale_factor=-1  dbl_ovrd=off  block_type=scale
      settings: infoedit=Scales input by a power of two by adjusting the binary point position.<P><P>Hardware notes: In hardware this block costs nothing.  block_version=VER_STRING_GOES_HERE
  Stage_UD : Subsystem
  RESET : Outport
  g_RF : Outport  Port=2
  g_BB : Outport  Port=3
  DONE : Outport  Port=4
  I_OUT : Outport  Port=5
  Q_OUT : Outport  Port=6
  wires:
  [TIMING] -> Stage_UD/3(Timing)
  [THRESHOLDS] -> RF_setting/4(Thresholds)
  Stage_UD/6(TOreset) -> Logical/1
  RF_setting/1(TOOLOW) -> Logical/2
  Logical/1 -> RESET/1
  RF_setting/3(RSSI_lock) -> BB_setting/4(RSSI_est)
  [EN_DCO_SUB] -> DCO_correction/8(EN_SUB)
  [DCO_Mode] -> DCO_correction/7(DCO_Mode)
  [DONE] -> DCO_correction/5(LOCKED)
  [RST] -> DCO_correction/3(RESET)
  Convert1/1 -> g_RF/1
  Convert/1 -> g_BB/1
  Scale/1 -> Convert/1
  DCO_correction/2(Q Out) -> Q_OUT/1
  DCO_correction/1(I Out) -> I_OUT/1
  Stage_UD/4(Stage0) -> RF_setting/1(EN)
  Stage_UD/3(Stage1) -> BB_setting/1(EN)
  RF_setting/2(G_RF) -> Convert1/1, BB_setting/3(G_RF)
  BB_setting/1(G_BB_est) -> Finalize_gBB/3(g_BB)
  Stage_UD/2(Stage2) -> Finalize_gBB/1(EN)
  RST/1 -> [RST], Stage_UD/2(Reset), BB_setting/2(RST), Finalize_gBB/2(RST), RF_setting/2(RST)
  EN/1 -> Stage_UD/1(EN)
  I_IN/1 -> DCO_correction/1(I in)
  Q_IN/1 -> DCO_correction/2(Q in)
  M_RST/1 -> DCO_correction/4(M_RESET)
  RSSI_dB/1 -> RF_setting/3(RSSI_IN)
  Stage_UD/1(Stage3) -> DONE/1, [DONE]
  Finalize_gBB/1(g_BB_out) -> Scale/1
  VIQ_IN/1 -> Finalize_gBB/6(VIQ)
  [ADJ_1] -> BB_setting/5(ADJ)
  [ADJ_2] -> Finalize_gBB/5(ADJ)
  [GBB_INIT] -> BB_setting/6(GBB_init)
  [T_dB] -> BB_setting/7(T_dB)
  [T_dB] -> Finalize_gBB/4(T_dB)
  [DCO_TIMING] -> DCO_correction/6(DCOTiming)

== system ofdm_agc_mimo/Control_System ==
  note: RESET_IN is passed through immediately and unblocks ENABLE one cycle later.
      |
      | PAKDET_IN triggers EN_HI, provided that neither RESET_IN nor M_RESET are asserted.
      | EN_HI is held hi until the next reset
      |
      | M_RESET asserts M_RESET_OUT and RESET for 100 cycles, and then unblocks the
      | EN port at the end of the 100 cycles
  note: confirmed
  RESET_IN : Inport
  M_RESET : Inport  Port=2
  PAKDET_IN : Inport  Port=3
  Delay2 : xbsIndex_r4/Delay  rst=off  infoeditControl=Selection of Reset will increase slice count due to use of real FFs and instead of SRLs  en=off  latency=1  dbl_ovrd=off  reg_retiming=off  block_type=delay
      settings: infoedit=Hardware notes: A delay line is a chain, each link of which is an SRL16 followed by a flip-flop. If register retiming is enabled, the delay line is a chain of flip-flops.  xl_area=[1 1 0 0 0 0 0]  block_version=VER_STRING_GOES_HERE
  EN_blocking : Subsystem
  Inverter : xbsIndex_r4/Inverter  en=off  latency=0  dbl_ovrd=off  block_type=inv
      settings: xl_area=[0 0 0 0 0 0 0]  block_version=VER_STRING_GOES_HERE
  Inverter1 : xbsIndex_r4/Inverter  en=off  latency=0  dbl_ovrd=off  block_type=inv
      settings: xl_area=[0 0 0 0 0 0 0]  block_version=VER_STRING_GOES_HERE
  Logical : xbsIndex_r4/Logical  logical_function=OR  inputs=2  en=off  latency=0  precision=Full  arith_type=Unsigned  n_bits=16  bin_pt=0  align_bp=on  dbl_ovrd=off  block_type=logical
      settings: xl_area=[1 0 0 1 0 0 0]  block_version=VER_STRING_GOES_HERE
  Logical1 : xbsIndex_r4/Logical  logical_function=AND  inputs=3  en=off  latency=0  precision=Full  arith_type=Unsigned  n_bits=16  bin_pt=0  align_bp=on  dbl_ovrd=off  block_type=logical
      settings: xl_area=[1 0 0 1 0 0 0]  block_version=VER_STRING_GOES_HERE
  Logical2 : xbsIndex_r4/Logical  logical_function=OR  inputs=2  en=off  latency=0  precision=Full  arith_type=Unsigned  n_bits=16  bin_pt=0  align_bp=on  dbl_ovrd=off  block_type=logical
      settings: xl_area=[1 0 0 1 0 0 0]  block_version=VER_STRING_GOES_HERE
  M_RESET_CTRL : Subsystem
  RisingEdge : Subsystem
  RisingEdge1 : Subsystem
  RisingEdge2 : Subsystem
  EN_HI : Outport
  RESET : Outport  Port=2
  M_RESET_OUT : Outport  Port=3
  wires:
  Delay2/1 -> Logical2/1
  Logical2/1 -> RESET/1
  RisingEdge1/1(Edge) -> Logical1/2
  Logical1/1 -> EN_blocking/1(EN_IN)
  Logical/1 -> EN_blocking/2(RESET)
  Inverter1/1 -> Logical1/3
  Inverter/1 -> Logical1/1
  RESET_IN/1 -> RisingEdge/1(IN), Inverter/1
  PAKDET_IN/1 -> RisingEdge1/1(IN)
  M_RESET/1 -> RisingEdge2/1(IN)
  RisingEdge2/1(Edge) -> M_RESET_CTRL/1(M_RESET)
  M_RESET_CTRL/2(M_RESET_OUT) -> Logical2/2, M_RESET_OUT/1, Inverter1/1
  EN_blocking/1(EN_blocked) -> EN_HI/1
  RisingEdge/1(Edge) -> Delay2/1, Logical/1
  M_RESET_CTRL/1(UNBLOCK_EN) -> Logical/2

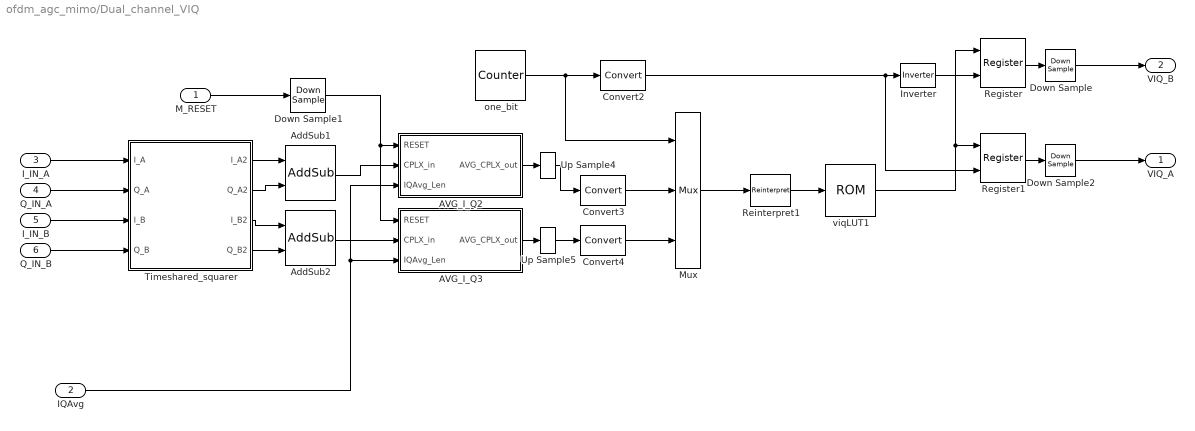
== system ofdm_agc_mimo/Dual_channel_VIQ ==
  M_RESET : Inport
  IQAvg : Inport  Port=2
  I_IN_A : Inport  Port=3
  Q_IN_A : Inport  Port=4
  I_IN_B : Inport  Port=5
  Q_IN_B : Inport  Port=6
  AVG_I_Q2 : Subsystem
  AVG_I_Q3 : Subsystem
  AddSub1 : xbsIndex_r4/AddSub  mode=Addition  use_carryin=off  use_carryout=off  en=off  latency=0  precision=Full  arith_type=Unsigned  n_bits=16  bin_pt=14  quantization=Truncate  overflow=Saturate  dbl_ovrd=off  use_behavioral_HDL=on  hw_selection=Fabric  pipelined=off  use_rpm=on  block_type=addsub
      settings: xl_area=[9 0 0 17 0 0 0]  block_version=VER_STRING_GOES_HERE
  AddSub2 : xbsIndex_r4/AddSub  mode=Addition  use_carryin=off  use_carryout=off  en=off  latency=0  precision=Full  arith_type=Unsigned  n_bits=16  bin_pt=14  quantization=Truncate  overflow=Saturate  dbl_ovrd=off  use_behavioral_HDL=on  hw_selection=Fabric  pipelined=off  use_rpm=on  block_type=addsub
      settings: xl_area=[9 0 0 17 0 0 0]  block_version=VER_STRING_GOES_HERE
  Convert2 : xbsIndex_r4/Convert  gui_display_data_type=Fixed-point  arith_type=Boolean  n_bits=11  bin_pt=10  float_type=Single  exp_bits=8  fraction_bits=24  quantization="Round  (unbiased: +/- Inf)"  overflow=Saturate  en=off  latency=0  dbl_ovrd=off  pipeline=off  block_type=convert
      settings: xl_area=[0 0 0 0 0 0 0]  block_version=VER_STRING_GOES_HERE
  Convert3 : xbsIndex_r4/Convert  gui_display_data_type=Fixed-point  arith_type=Unsigned  n_bits=11  bin_pt=10  float_type=Single  exp_bits=8  fraction_bits=24  quantization="Round  (unbiased: +/- Inf)"  overflow=Saturate  en=off  latency=0  dbl_ovrd=off  pipeline=off  block_type=convert
      settings: xl_area=[14 0 0 27 0 0 0]  block_version=VER_STRING_GOES_HERE
  Convert4 : xbsIndex_r4/Convert  gui_display_data_type=Fixed-point  arith_type=Unsigned  n_bits=11  bin_pt=10  float_type=Single  exp_bits=8  fraction_bits=24  quantization="Round  (unbiased: +/- Inf)"  overflow=Saturate  en=off  latency=0  dbl_ovrd=off  pipeline=off  block_type=convert
      settings: xl_area=[14 0 0 27 0 0 0]  block_version=VER_STRING_GOES_HERE
  Down Sample : xbsIndex_r4/Down Sample  sample_ratio=2  sample_phase="Last Value of Frame  (most efficient)"  en=off  latency=1  dbl_ovrd=off  block_type=dsamp
      settings: xl_area=[5 9 0 0 0 0 0]  block_version=VER_STRING_GOES_HERE
  Down Sample1 : xbsIndex_r4/Down Sample  sample_ratio=4  sample_phase="Last Value of Frame  (most efficient)"  en=off  latency=1  dbl_ovrd=off  block_type=dsamp
      settings: xl_area=[1 1 0 0 0 0 0]  block_version=VER_STRING_GOES_HERE
  Down Sample2 : xbsIndex_r4/Down Sample  sample_ratio=2  sample_phase="Last Value of Frame  (most efficient)"  en=off  latency=1  dbl_ovrd=off  block_type=dsamp
      settings: xl_area=[5 9 0 0 0 0 0]  block_version=VER_STRING_GOES_HERE
  Inverter : xbsIndex_r4/Inverter  en=off  latency=0  dbl_ovrd=off  block_type=inv
      settings: xl_area=[0 0 0 0 0 0 0]  block_version=VER_STRING_GOES_HERE
  Mux : xbsIndex_r4/Mux  inputs=2  en=off  latency=0  precision=Full  arith_type=Unsigned  n_bits=16  bin_pt=14  quantization=Truncate  overflow=Wrap  dbl_ovrd=off  block_type=mux
      settings: xl_area=[6 0 0 11 0 0 0]  block_version=VER_STRING_GOES_HERE
  Register : xbsIndex_r4/Register  init=0  rst=off  en=on  dbl_ovrd=off  block_type=register
      settings: xl_area=[5 9 0 0 0 0 0]  block_version=VER_STRING_GOES_HERE
  Register1 : xbsIndex_r4/Register  init=0  rst=off  en=on  dbl_ovrd=off  block_type=register
      settings: xl_area=[5 9 0 0 0 0 0]  block_version=VER_STRING_GOES_HERE
  Reinterpret1 : xbsIndex_r4/Reinterpret  force_arith_type=off  arith_type=Unsigned  force_bin_pt=on  bin_pt=0  block_type=cast
      settings: infoedit="Changes type of samples without altering their binary representation.<P><P>Hardware notes: In hardware this block costs nothing.<P><P>Example:  Suppose the input is 6 bits wide, signed, with 2 fractional bits, and the output is forced to unsigned with 0 fractional bits.  Then an input of -2.0 (1110.00 in binary 2's complement) becomes an output of 56 (111000 in binary)."  block_version=VER_STRING_GOES_HERE
  Timeshared_squarer : Subsystem
  Up Sample4 : xbsIndex_r4/Up Sample  sample_ratio=2  copy_samples=on  en=off  latency=0  dbl_ovrd=off  block_type=usamp
      settings: infoedit="Up samples input data.  Inserted values  can be zeros or copies of the most recent input sample.<P><P>Hardware notes: No hardware is needed if inserted values are copies of the input sample; otherwise, a mux and single bit flip-flop are used."  xl_area=[0 0 0 0 0 0 0]  block_version=VER_STRING_GOES_HERE
  Up Sample5 : xbsIndex_r4/Up Sample  sample_ratio=2  copy_samples=on  en=off  latency=0  dbl_ovrd=off  block_type=usamp
      settings: infoedit="Up samples input data.  Inserted values  can be zeros or copies of the most recent input sample.<P><P>Hardware notes: No hardware is needed if inserted values are copies of the input sample; otherwise, a mux and single bit flip-flop are used."  xl_area=[0 0 0 0 0 0 0]  block_version=VER_STRING_GOES_HERE
  one_bit : xbsIndex_r4/Counter  cnt_type=Free Running  cnt_to=Inf  operation=Up  start_count=0  cnt_by_val=1  arith_type=Unsigned  n_bits=1  bin_pt=0  load_pin=off  rst=off  en=off  explicit_period=on  period=1  dbl_ovrd=off  use_behavioral_HDL=off  implementation=Fabric  use_rpm=off  block_type=counter
      settings: xl_area=[2 1 0 1 0 0 0]  block_version=VER_STRING_GOES_HERE
  viqLUT1 : xbsIndex_r4/ROM  depth=2^11  initVector=20*log10(sqrt(ltbl))  distributed_mem=Block RAM  rst=off  init_reg=0  en=off  latency=1  gui_display_data_type=Fixed-point  arith_type="Signed  (2's comp)"  n_bits=9  bin_pt=2  preci_type=Single  exp_width=8  frac_width=24  dbl_ovrd=off  optimize=Area  use_rpm=off  block_type=sprom
      settings: xl_area=[79 9 0 158 0 0 0]  block_version=VER_STRING_GOES_HERE
  VIQ_A : Outport
  VIQ_B : Outport  Port=2
  wires:
  Q_IN_B/1 -> Timeshared_squarer/4(Q_B)
  I_IN_B/1 -> Timeshared_squarer/3(I_B)
  Q_IN_A/1 -> Timeshared_squarer/2(Q_A)
  I_IN_A/1 -> Timeshared_squarer/1(I_A)
  Reinterpret1/1 -> viqLUT1/1
  Convert2/1 -> Inverter/1, Register1/2
  Up Sample5/1 -> Convert4/1
  Up Sample4/1 -> Convert3/1
  Down Sample2/1 -> VIQ_A/1
  Down Sample/1 -> VIQ_B/1
  Register/1 -> Down Sample/1
  Register1/1 -> Down Sample2/1
  Inverter/1 -> Register/2
  viqLUT1/1 -> Register1/1, Register/1
  Mux/1 -> Reinterpret1/1
  Convert4/1 -> Mux/3
  Convert3/1 -> Mux/2
  one_bit/1 -> Convert2/1, Mux/1
  AVG_I_Q3/1(AVG_CPLX_out) -> Up Sample5/1
  AVG_I_Q2/1(AVG_CPLX_out) -> Up Sample4/1
  Down Sample1/1 -> AVG_I_Q2/1(RESET), AVG_I_Q3/1(RESET)
  M_RESET/1 -> Down Sample1/1
  AddSub1/1 -> AVG_I_Q2/2(CPLX_in)
  AddSub2/1 -> AVG_I_Q3/2(CPLX_in)
  Timeshared_squarer/4(Q_B2) -> AddSub2/2
  Timeshared_squarer/3(I_B2) -> AddSub2/1
  Timeshared_squarer/2(Q_A2) -> AddSub1/2
  Timeshared_squarer/1(I_A2) -> AddSub1/1
  IQAvg/1 -> AVG_I_Q2/3(IQAvg_Len), AVG_I_Q3/3(IQAvg_Len)
